simulink model "Elivator"  (R2024b)
settings: Solver=VariableStepAuto  StartTime=0.0  StopTime=inf  RelTol=1e-3
settings Model: Creator=ksamb  LastModifiedBy=ksamb

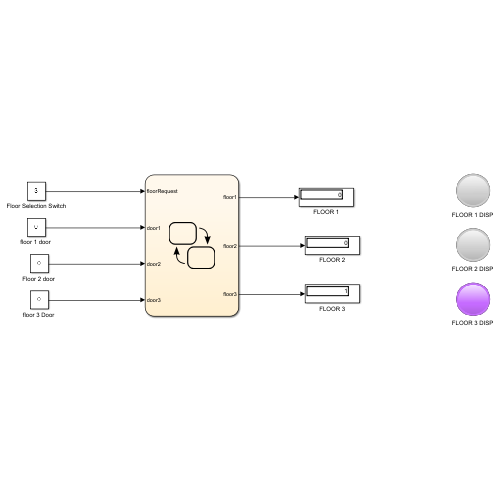
[thumbnail: Simulink's stored preview of the top-level diagram]
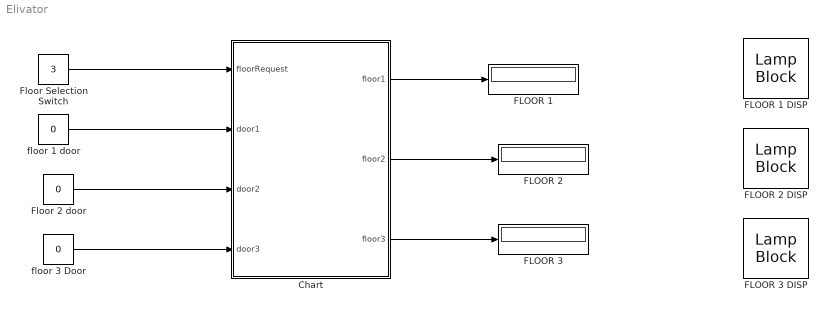
== system Elivator ==
  Chart : Stateflow chart  TreatAsAtomicUnit=on
  FLOOR 1 : Display
  FLOOR 1 DISP : LampBlock  LabelPosition=Hide
  FLOOR 2 : Display
  FLOOR 2 DISP : LampBlock  LabelPosition=Hide
  FLOOR 3 : Display
  FLOOR 3 DISP : LampBlock  LabelPosition=Hide
  "Floor 2 door " : Constant  Value=0
  Floor Selection Switch : Constant  Value=3
  "floor 1 door " : Constant  Value=0
  "floor 3 Door " : Constant  Value=0
  wires:
  Floor Selection Switch/1 -> Chart/1(floorRequest)
  "floor 3 Door "/1 -> Chart/4(door3)
  "Floor 2 door "/1 -> Chart/3(door2)
  "floor 1 door "/1 -> Chart/2(door1)
  Chart/2(floor2) -> FLOOR 2/1
  Chart/1(floor1) -> FLOOR 1/1
  Chart/3(floor3) -> FLOOR 3/1

== stateflow chart Elivator/Chart ==
  state FLOOR1
    state DoorClose
      entry:
      door1==0;
      door1==1
      floor1=1;
      floor2=0;
      floor3=0;
    (default) -> FLOOR1.DoorClose
  state FLOOR2
    state DoorClose
      entry:
      door2==0;
      door2==1;
      floor2=1;
      floor3=0;
      floor1=0;
    (default) -> FLOOR2.DoorClose
  state FLOOR3
    state DoorClose
      entry:
      door3==0;
      door3==1;
      floor3=1;
      floor2=0;
      floor1=0;
    (default) -> FLOOR3.DoorClose
  FLOOR1 -> FLOOR3 [order 2] : [floorRequest == 3 && door1==0 && door2==0 && door1==0]
  (default) -> FLOOR1
  FLOOR1 -> FLOOR2 [order 1] : [floorRequest == 2 &&...
      | door1==0 &&...
      | door3==0 && door2==0]
  FLOOR2 -> FLOOR3 [order 2] : [floorRequest == 3 &&...
      |  door2==0 &&...
      | door3==0 && door1==0]
  FLOOR2 -> FLOOR1 [order 1] : [floorRequest == 1 &&...
      |  door2==0 &&...
      | door3==0 && door1==0]
  FLOOR3 -> FLOOR2 [order 1] : [floorRequest == 2 && door3==0&&...
      | door2==0 && door1==0]
  FLOOR3 -> FLOOR1 [order 2] : [floorRequest == 1 &&...
      |  door3==0 &&...
      | door2==0 && door1==0]
  data: floorRequest input; door1 input; door2 input; door3 input; floor1 output; floor2 output; floor3 output
